simulink model "Operative_control"  (R2023a)
settings: Solver=VariableStepAuto  StartTime=0.0  StopTime=30  RelTol=1e-6  AbsTol=1e-6
undefined symbols (not defined in the file): DiscIntNeverNeededParam, f_s, Kd_op, Ki_op, Kp_op
settings Model: Creator=Angelo  LastModifiedBy=Savio Del Peschio
settings OptimizationCC: ReuseModelBlockBuffer=off
settings DebuggingCC: UnconnectedInputMsg=warning  UnconnectedOutputMsg=warning  UnconnectedLineMsg=warning
settings ModelReferenceCC: EnableRefExpFcnMdlSchedulingChecks=on
settings RTWCC: DLArmComputeVersion=19.05

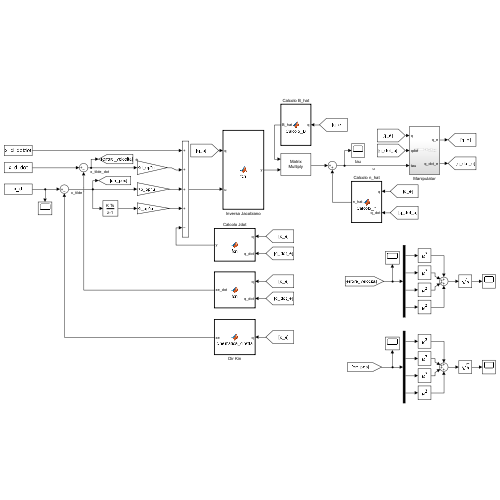
[thumbnail: Simulink's stored preview of the top-level diagram]
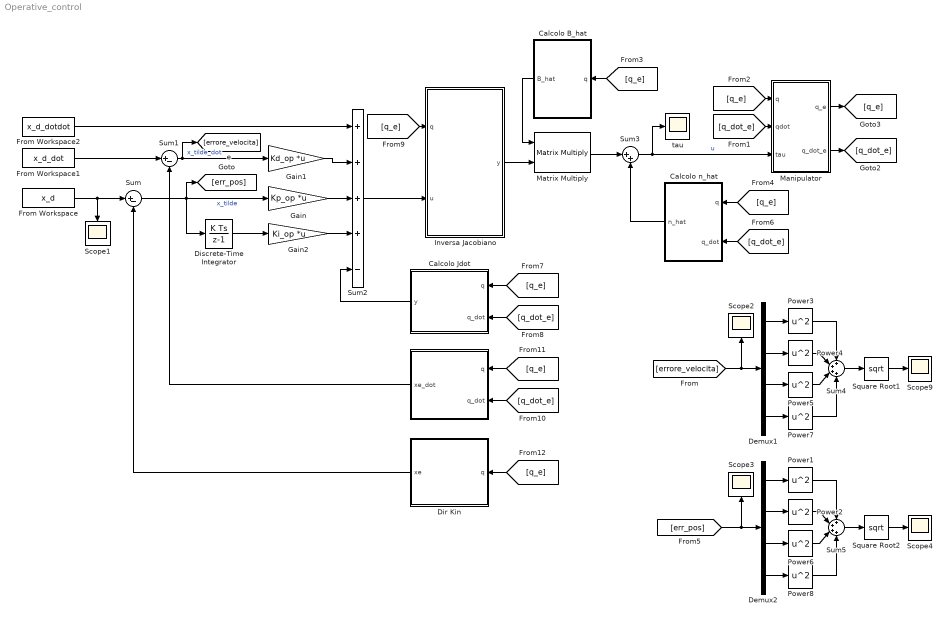
== system Operative_control ==
  " " : MATLAB Function  TreatAsAtomicUnit=on
  Calcolo B_hat : MATLAB Function  TreatAsAtomicUnit=on
  Calcolo Jdot : MATLAB Function  TreatAsAtomicUnit=on
  Calcolo n_hat : MATLAB Function  TreatAsAtomicUnit=on
  Demux1 : Demux
  Demux2 : Demux
  Dir Kin : MATLAB Function  TreatAsAtomicUnit=on
  Discrete-Time Integrator : DiscreteIntegrator  InitialCondition=zeros(4,1)  SampleTime=1/f_s  ICPrevOutput=DiscIntNeverNeededParam  ICPrevScaledInput=DiscIntNeverNeededParam
  From Workspace : FromWorkspace  VariableName=x_d  SampleTime=1/f_s  OutputAfterFinalValue=Holding final value
  From Workspace1 : FromWorkspace  VariableName=x_d_dot  SampleTime=1/f_s  OutputAfterFinalValue=Setting to zero
  From Workspace2 : FromWorkspace  VariableName=x_d_dotdot  SampleTime=1/f_s  OutputAfterFinalValue=Setting to zero
  Gain : Gain  Gain=Kp_op  Multiplication=Matrix(K*u)
  Gain1 : Gain  Gain=Kd_op  Multiplication=Matrix(K*u)
  Gain2 : Gain  Gain=Ki_op  Multiplication=Matrix(K*u)
  "Inversa Jacobiano " : MATLAB Function  TreatAsAtomicUnit=on
  Manipulator : Subsystem
  Matrix Multiply : Product  Multiplication=Matrix(*)
  Power{1..8} (8 alike) : Math  Operator=square
  Scope{1..4,9} (5 alike) : Scope
  Square Root1 : Sqrt
  Square Root2 : Sqrt
  Sum : Sum  Inputs=|+-
  Sum1 : Sum  Inputs=|+-
  Sum2 : Sum  Inputs=++++-
  Sum3 : Sum  Inputs=|++
  Sum4 : Sum  Inputs=++++
  Sum5 : Sum  Inputs=++++
  tau : Scope
  wires:
  From Workspace1/1 -> Sum1/1
  Sum/1 -> Gain/1, [err_pos], Discrete-Time Integrator/1  "x_tilde"
  Sum1/1 -> [errore_velocita], Gain1/1  "x_tilde_dot"
  From Workspace2/1 -> Sum2/1
  Gain1/1 -> Sum2/2
  Sum2/1 -> "Inversa Jacobiano "/2(u)
  Calcolo B_hat/1(B_hat) -> Matrix Multiply/1
  "Inversa Jacobiano "/1(y) -> Matrix Multiply/2
  Manipulator/2(q_dot_e) -> [q_dot_e]
  Matrix Multiply/1 -> Sum3/1
  Sum3/1 -> tau/1, Manipulator/3(tau)  "u"
  Calcolo n_hat/1(n_hat) -> Sum3/2
  " "/1(xe_dot) -> Sum1/2
  Gain/1 -> Sum2/3
  Discrete-Time Integrator/1 -> Gain2/1
  Gain2/1 -> Sum2/4
  Calcolo Jdot/1(y) -> Sum2/5
  Dir Kin/1(xe) -> Sum/2
  [errore_velocita] -> Scope2/1, Demux1/1
  Power3/1 -> Sum4/1
  Sum4/1 -> Square Root1/1
  Power4/1 -> Sum4/2
  Demux1/2 -> Power4/1
  Demux1/1 -> Power3/1
  Power5/1 -> Sum4/3
  Demux1/3 -> Power5/1
  Square Root1/1 -> Scope9/1
  From Workspace/1 -> Sum/1, Scope1/1
  Demux1/4 -> Power7/1
  [q_dot_e] -> Manipulator/2(qdot)
  Manipulator/1(q_e) -> [q_e]
  [q_e] -> Manipulator/1(q)
  [q_e] -> Calcolo B_hat/1(q)
  [q_e] -> Calcolo n_hat/1(q)
  [q_dot_e] -> Calcolo n_hat/2(q_dot)
  [q_e] -> Calcolo Jdot/1(q)
  [q_dot_e] -> Calcolo Jdot/2(q_dot)
  [q_dot_e] -> " "/2(q_dot)
  [q_e] -> " "/1(q)
  [q_e] -> Dir Kin/1(q)
  Power7/1 -> Sum4/4
  Power8/1 -> Sum5/4
  Demux2/4 -> Power8/1
  Square Root2/1 -> Scope4/1
  Power2/1 -> Sum5/2
  Power1/1 -> Sum5/1
  Sum5/1 -> Square Root2/1
  Demux2/2 -> Power2/1
  Demux2/1 -> Power1/1
  Demux2/3 -> Power6/1
  Power6/1 -> Sum5/3
  [err_pos] -> Scope3/1, Demux2/1
  [q_e] -> "Inversa Jacobiano "/1(q)

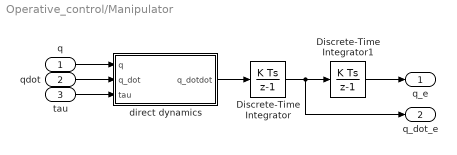
== system Operative_control/Manipulator ==
  q : Inport
  qdot : Inport  Port=2
  tau : Inport  Port=3
  Discrete-Time Integrator : DiscreteIntegrator  InitialCondition=zeros(4,1)  SampleTime=1/f_s  ICPrevOutput=DiscIntNeverNeededParam  ICPrevScaledInput=DiscIntNeverNeededParam
  Discrete-Time Integrator1 : DiscreteIntegrator  InitialCondition=config_p_init'  SampleTime=1/f_s  ICPrevOutput=DiscIntNeverNeededParam  ICPrevScaledInput=DiscIntNeverNeededParam
  direct dynamics : MATLAB Function  TreatAsAtomicUnit=on
  q_e : Outport
  q_dot_e : Outport  Port=2
  wires:
  tau/1 -> direct dynamics/3(tau)
  q/1 -> direct dynamics/1(q)
  Discrete-Time Integrator1/1 -> q_e/1
  qdot/1 -> direct dynamics/2(q_dot)
  Discrete-Time Integrator/1 -> q_dot_e/1, Discrete-Time Integrator1/1
  direct dynamics/1(q_dotdot) -> Discrete-Time Integrator/1

== matlab function Operative_control/Inversa Jacobiano  ==
  data: q input; y output; u input
function y = fcn(q,u)

    J = [-0.5*sin(q(1))-0.5*sin(q(1)+q(2))   -0.5*sin(q(1)+q(2))    0  0 
          0.5*cos(q(1))+0.5*cos(q(1)+q(2))    0.5*cos(q(1)+q(2))    0  0 
          0                                   0                    -1  0
          1                                   1                     0  -1];
    
    y = inv(J)*u;

end

== matlab function Operative_control/  ==
  data: q input; xe_dot output; q_dot input
function xe_dot= fcn(q, q_dot)

    J = [-0.5*sin(q(1))-0.5*sin(q(1)+q(2))   -0.5*sin(q(1)+q(2))    0  0 
          0.5*cos(q(1))+0.5*cos(q(1)+q(2))    0.5*cos(q(1)+q(2))    0  0 
          0                                   0                    -1  0
          1                                   1                     0  -1];

    xe_dot = J*q_dot;

end

== matlab function Operative_control/Calcolo Jdot ==
  data: q input; q_dot input; y output
function y = fcn(q, q_dot)

    J_dot = [-0.5*(q_dot(1)+q_dot(2))*cos(q(1)+q(2))-0.5*q_dot(1)*cos(q(1))              -0.5*(q_dot(1)+q_dot(2))*cos(q(1)+q(2))  0   0
             -0.5*(q_dot(1)+q_dot(2))*sin(q(1)+q(2))-0.5*q_dot(1)*sin(q(1))              -0.5*(q_dot(1)+q_dot(2))*sin(q(1)+q(2))  0   0
             0                                                                            0                                       0   0
             0                                                                            0                                       0   0];

    y = J_dot*q_dot;

end

== matlab function Operative_control/Manipulator/direct dynamics ==
  data: q input; q_dot input; q_dotdot output; tau input
function q_dotdot = fcn(q, q_dot, tau)
       
    %attriti dei motori
    Fm1 = 0.00005;
    Fm2 = 0.00005;
    Fm3 = 0.01;
    Fm4 = 0.005;
    
    theta_2 = q(2);
    theta_dot_1 = q_dot(1);
    theta_dot_2 = q_dot(2);
    d_dot_3 = q_dot(3);
    theta_dot_4 = q_dot(4);
    
    B_p = [(25*cos(theta_2))/2 + 12013/500, (25*cos(theta_2))/4 + 1252/125, -1/4, -51/50;
            (25*cos(theta_2))/4 + 1252/125,                       1252/125, -1/4, -51/50;
                                      -1/4,                           -1/4, 55/2,      0;
                                    -51/50,                         -51/50,    0,    7/5];                                                                                                        
       
    C_p = [-(25*theta_dot_2*sin(theta_2))/4, - (25*theta_dot_1*sin(theta_2))/4 - (25*theta_dot_2*sin(theta_2))/4, 0, 0;
            (25*theta_dot_1*sin(theta_2))/4,                                                                   0, 0, 0;
                                          0,                                                                   0, 0, 0;
                                          0,                                                                   0, 0, 0];
    
    
    Fv = diag([-Fm1 -Fm2 -Fm3 -Fm4]);
    g = [0, 0, - 9.81*(5+10), 0]';
    tau_primo = C_p*q_dot+Fv*q_dot+g;
    
    q_dotdot = inv(B_p)*(tau-tau_primo); 

end

== matlab function Operative_control/Dir Kin ==
  data: q input; xe output
function xe = cinematica_diretta(q)
    
    xe = [  0.5*cos(q(1))+0.5*cos(q(1)+q(2));
            0.5*sin(q(1))+0.5*sin(q(1)+q(2));
            1/2-q(3)
            q(1)+q(2)-q(4) ];

end

== matlab function Operative_control/Calcolo B_hat ==
  data: q input; B_hat output
function B_hat = Calcolo_B(q)

    theta_1 = q(1);
    theta_2 = q(1);
    d_3 = q(1);
    theta_4 = q(1);

    B_hat = [10*cos(theta_2) + 10763/500, 5*cos(theta_2) + 4383/500, -1/4, -51/50;
             5*cos(theta_2) + 4383/500,                  4383/500, -1/4, -51/50;
                                  -1/4,                      -1/4, 45/2,      0;
                                -51/50,                    -51/50,    0,    7/5];

end

== matlab function Operative_control/Calcolo n_hat ==
  data: q input size=[4]; n_hat output; q_dot input
function n_hat = Calcolo_n(q, q_dot)

    % attriti dei motori
    Fm1 = 0.00005;
    Fm2 = 0.00005;
    Fm3 = 0.01;
    Fm4 = 0.005;
    
    theta_1 = q(1);
    theta_2 = q(2);
    d_3 = q(3);
    theta_4 = q(4);
    theta_dot_1 = q_dot(1);
    theta_dot_2 = q_dot(2);
    
    C = [-5*theta_dot_2*sin(theta_2), -5*theta_dot_1*sin(theta_2) - 5*theta_dot_2*sin(theta_2), 0, 0;
          5*theta_dot_1*sin(theta_2), 0,                                                        0, 0;
          0,                          0,                                                        0, 0;
          0,                          0,                                                        0, 0];
    
    Fv = diag([-Fm1 -Fm2 -Fm3 -Fm4]);
    
    g = [0, 0, -9.81*10, 0]';
    
    n_hat= C*q_dot+Fv*q_dot+g;

end
